simulink subsystem "SIM_DZ"  (R2023a)
settings: Solver=VariableStepAuto  StartTime=0.0  StopTime=10.0  RelTol=1e-3
settings Model: Creator=ycheb  LastModifiedBy=ycheb

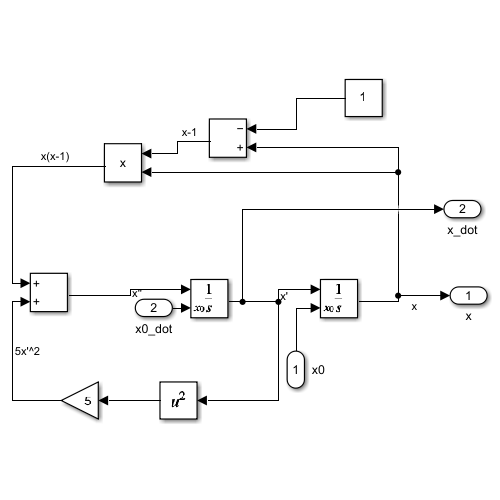
[thumbnail: Simulink's stored preview of the top-level diagram]
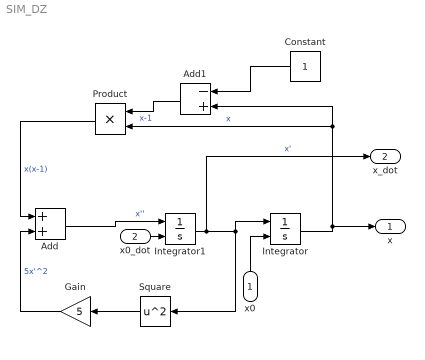
== system SIM_DZ ==
  x0 : Inport
  x0_dot : Inport  Port=2
  Add : Sum
  Add1 : Sum  Inputs=-+
  Constant : Constant
  Gain : Gain  Gain=5
  Integrator : Integrator  InitialConditionSource=external
  Integrator1 : Integrator  InitialConditionSource=external
  Product : Product
  Square : Math  Operator=square
  x : Outport
  x_dot : Outport  Port=2
  wires:
  Integrator1/1 -> Square/1, Integrator/1, x_dot/1  "x'"
  Integrator/1 -> x/1, Add1/2, Product/2  "x"
  Add/1 -> Integrator1/1  "x''"
  Square/1 -> Gain/1
  Gain/1 -> Add/2  "5x'^2"
  Constant/1 -> Add1/1
  Add1/1 -> Product/1  "x-1"
  Product/1 -> Add/1  "x(x-1)"
  x0_dot/1 -> Integrator1/2
  x0/1 -> Integrator/2
